simulink model "AGI_hydrogen_test9"  (R2024b)
settings: Solver=VariableStepAuto  StartTime=0.0  StopTime=Test.t_sim  RelTol=1e-3
values from neighbouring files (symbols this model uses):
  ControlSampleTime = 1/8000    (= 0.000125)    [init.m]
  f_Batt_ref = [46 47 49.9 50.1 52 53]    [init.m]
  f_PV_ref = [46 50.1 52 53]    [init.m]
  Hy_current_Ki = 20    [init.m]
  Hy_current_Kp = 0.3    [init.m]
  P_Batt_ref = [0.5 0.5 0 0 -0.5 -0.5]    [init.m]
  P_PV_ref = [1 1 1 1]    [init.m]
  PLL_Ki = 100    [init.m]
  PLL_Kp = 30    [init.m]
  Q_Batt_ref = [-0.5 -0.5 0 0.5 0.5]    [init.m]
  Q_PV_ref = [-0.5 -0.5 0 0.5 0.5]    [init.m]
  Q_ref_pu_VSM = 1    [init.m]
  S_AGI = SC_AGI    (= 25000)    [init.m]
  Test =     [S-Rocof1-OC1.mat]    (also in S-VolAngStep4-OC1.mat)
  Ts = ControlSampleTime    (= 0.000125)    [init.m]
  Ts_Control = 1e-4    (= 0.0001)    [init.m]
  Ts_Power = 5e-5    (= 5e-05)    [init.m]
  U_Batt_ref = [0.8 0.9 1 1.1 1.2]    [init.m]
  U_PV_ref = [0.8 0.9 1 1.1 1.2]    [init.m]
undefined symbols (not defined in the file or in its folder): DiscIntNeverNeededParam, Grid, Ion, L_line_PV, LCL, Lithium, sps, VSMCTRL
libraries: spsThreePhaseSeriesRLCBranchLib x10, powerlib_extras x9, spsSeriesRLCBranchLib x8, spsThreePhaseVIMeasurementLib x6, spsThreePhaseBreakerLib x6, slpidlib x6, simulink x6, spsVoltageMeasurementLib x6, FriedrichLibrary x6, spsPowerPositiveSequenceLib x5, spsUniversalBridgeLib x4, spsControlledVoltageSourceLib x4
(part 1 of 3)
settings Model: Creator=e2n051  LastModifiedBy=wshan
settings RTWCC: GPUComputeCapability=3.5

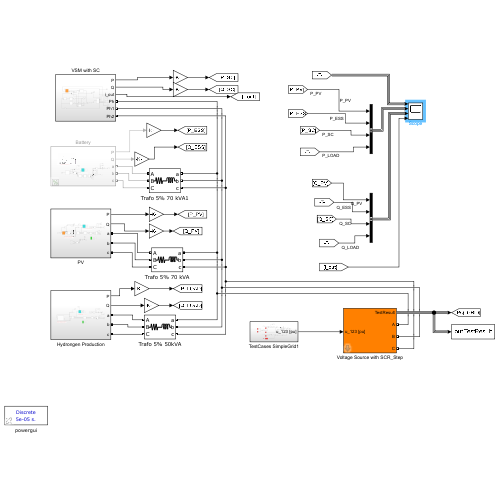
[thumbnail: Simulink's stored preview of the top-level diagram]
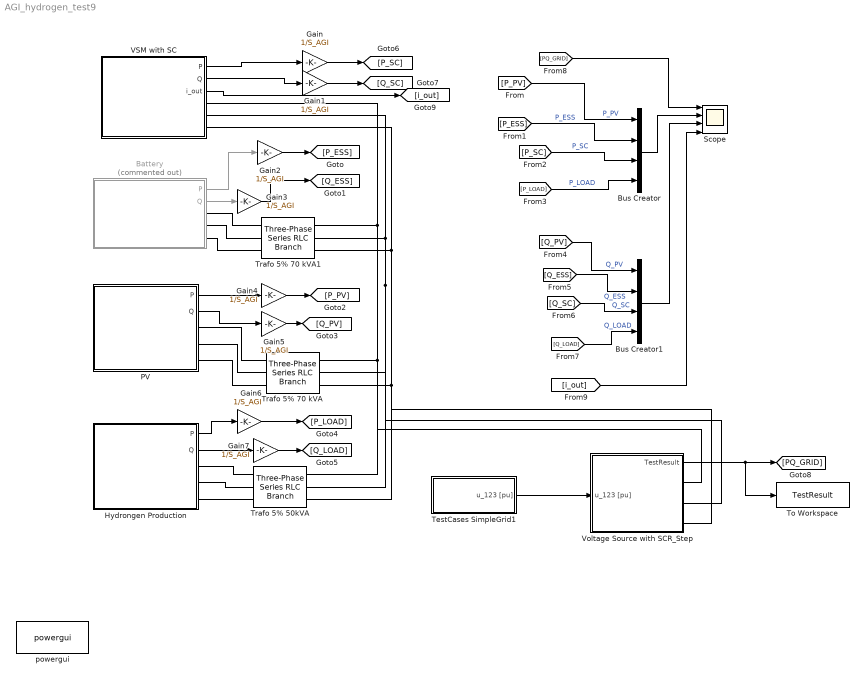
== system AGI_hydrogen_test9 ==
  Battery : Subsystem  Commented=on
  Bus Creator : BusCreator  Inputs=4
  Bus Creator1 : BusCreator  Inputs=4
  Gain{,1..7} (8 alike) : Gain  Gain=1/S_AGI
  Hydrongen Production : Subsystem
  PV : Subsystem
  Scope : Scope  NumInputPorts=4
  TestCases SimpleGrid1 : Subsystem
  To Workspace : ToWorkspace  VariableName=TestResult  SaveFormat=Timeseries  SampleTime=-1
  Trafo 5% 50kVA : spsThreePhaseSeriesRLCBranchLib/Three-Phase Series RLC Branch  LConnTagsString=A|B|C  RConnTagsString=A|B|C  BranchType=RL  Resistance=1e-3  Inductance=Test.x_trafo_pu*(400^2/(50e3))/(2*pi*50)  Capacitance=inf  Measurements=None
  Trafo 5% 70 kVA : spsThreePhaseSeriesRLCBranchLib/Three-Phase Series RLC Branch  LConnTagsString=A|B|C  RConnTagsString=A|B|C  BranchType=RL  Resistance=1e-3  Inductance=Test.x_trafo_pu*(400^2/(70e3))/(2*pi*50)  Capacitance=inf  Measurements=None
  Trafo 5% 70 kVA1 : spsThreePhaseSeriesRLCBranchLib/Three-Phase Series RLC Branch  LConnTagsString=A|B|C  RConnTagsString=A|B|C  BranchType=RL  Resistance=1e-3  Inductance=Test.x_trafo_pu*(400^2/(70e3))/(2*pi*50)  Capacitance=inf  Measurements=None
  VSM with SC : Subsystem
  Voltage Source with SCR_Step : Subsystem  mask{f0=50, Vbase=400, Sbase=S_AGI, Lpu1=Test.x_grid1, Lpu2=Test.x_grid2, Rpu1=Test.r_grid1, Rpu2=Test.r_grid2, tstep=Test.t_xgrid}
      mask prompts: f0 "Nominal Grid Frequency in Hz"; Vbase "Vbase Ph-Ph in V"; Sbase "Sbase in VA"; Lpu1 "initial X_grid in p.u."; Lpu2 "final X_grid in p.u."; Rpu1 "initial R_grid in p.u."; Rpu2 "final R_grid in p.u."; tstep "Step time grid impedance in s"
  powergui : spspowerguiLib/powergui  Priority=1  SimulationMode=Discrete  SampleTime=Ts_Power  frequency=60  Iterations=50  frequencyindice=0  Pbase=100e6  ErrMax=1e-4  UnitsV=kV  UnitsW=MW  buscounter=0  FunctionMessages=off  echomessages=off  EnableUseOfTLC=off  CurrentSourceSwitches=off  DisableSnubberDevices=off  DisableRonSwitches=off  DisableVfSwitches=off  DisplayEquations=off  AutomaticDiscreteSolvers=off  SolverType=Tustin  Interpol=off  ExternalGateDelay=off  methode=off  Ts=0  x0status=blocks  SPID=off  SwTol=0  HookPort=off  NonlinearTolerance=1e-4  nMaxIteration=100  ContinueOnMaxIteration=off  RestoreLinks=warning  ResistiveCurrentMeasurement=off  Frange=[0:2:500]  Ylog=off  Xlog=on  ShowGrid=off  save=off  variable=ZData  structure=0  ZoomFFT=on  StartTime=0.0  cycles=1  DisplayStyle=1  fundamental=60  FreqAxis=off  MaxFrequency=1000  frequencyindicesteady=1  RmsSteady=1  display=off
  wires:
  Battery/1(P) -> Gain2/1
  Battery/2(Q) -> Gain3/1
  PV/2(Q) -> Gain5/1
  PV/1(P) -> Gain4/1
  Hydrongen Production/1(P) -> Gain6/1
  Hydrongen Production/2(Q) -> Gain7/1
  VSM with SC/1(P) -> Gain/1
  [P_ESS] -> Bus Creator/2  "P_ESS"
  [P_SC] -> Bus Creator/3  "P_SC"
  Bus Creator/1 -> Scope/2
  VSM with SC/2(Q) -> Gain1/1
  [P_LOAD] -> Bus Creator/4  "P_LOAD"
  [Q_ESS] -> Bus Creator1/2  "Q_ESS"
  [Q_SC] -> Bus Creator1/3  "Q_SC"
  Bus Creator1/1 -> Scope/3
  [Q_PV] -> Bus Creator1/1  "Q_PV"
  [Q_LOAD] -> Bus Creator1/4  "Q_LOAD"
  [PQ_GRID] -> Scope/1
  VSM with SC/3(i_out) -> [i_out]
  [i_out] -> Scope/4
  Voltage Source with SCR_Step/1(TestResult) -> To Workspace/1, [PQ_GRID]
  TestCases SimpleGrid1/1(u_123 [pu]) -> Voltage Source with SCR_Step/1(u_123 [pu])
  [P_PV] -> Bus Creator/1  "P_PV"
  Gain/1 -> [P_SC]
  Gain1/1 -> [Q_SC]
  Gain2/1 -> [P_ESS]
  Gain3/1 -> [Q_ESS]
  Gain4/1 -> [P_PV]
  Gain5/1 -> [Q_PV]
  Gain6/1 -> [P_LOAD]
  Gain7/1 -> [Q_LOAD]
  connections:
  Trafo 5% 70 kVA1/RConn1 -- Voltage Source with SCR_Step/RConn1 -- Trafo 5% 50kVA/RConn1 -- Trafo 5% 70 kVA/RConn1 -- VSM with SC/RConn1
  Trafo 5% 70 kVA1/RConn3 -- Voltage Source with SCR_Step/RConn3 -- Trafo 5% 50kVA/RConn3 -- Trafo 5% 70 kVA/RConn3 -- VSM with SC/RConn3
  Trafo 5% 70 kVA1/LConn3 -- Battery/RConn3
  Trafo 5% 70 kVA1/LConn1 -- Battery/RConn1
  Trafo 5% 70 kVA1/LConn2 -- Battery/RConn2
  PV/RConn1 -- Trafo 5% 70 kVA/LConn1
  PV/RConn2 -- Trafo 5% 70 kVA/LConn2
  PV/RConn3 -- Trafo 5% 70 kVA/LConn3
  Trafo 5% 70 kVA1/RConn2 -- Voltage Source with SCR_Step/RConn2 -- Trafo 5% 50kVA/RConn2 -- Trafo 5% 70 kVA/RConn2 -- VSM with SC/RConn2
  Hydrongen Production/RConn1 -- Trafo 5% 50kVA/LConn1
  Hydrongen Production/RConn2 -- Trafo 5% 50kVA/LConn2
  Hydrongen Production/RConn3 -- Trafo 5% 50kVA/LConn3

== system AGI_hydrogen_test9/Battery ==
  note: Simple Battery Model from Matlab Standard Library:
  note: q-u-static implemented inside DC-AC converter control
  Battery : spsBatteryLib/Battery  BatType=Lithium-Ion  NomV=720  NomQ=10000  SOC=80  Batt_Tr=30  PresetModel=on  MaxQ=10000  MinV=540  FullV=838.0707  Dis_rate=4347.8261  R=0.00072  Normal_OP=9043.4783  expZone="[777.8778      491.3043]"
  L : spsThreePhaseSeriesRLCBranchLib/Three-Phase Series RLC Branch  LConnTagsString=A|B|C  RConnTagsString=A|B|C  BranchType=RL  Resistance=1e-3  Inductance=45e-6  Capacitance=inf  Measurements=None
  Mux4 : Mux  Inputs=2
  Power (Positive-Sequence) : spsPowerPositiveSequenceLib/Power (Positive-Sequence)  Freq=50  Vinit=[20200 0]  Iinit=[12.3 0]  Ts=Ts_Control
  Scope{,1..4} (5 alike) : Scope
  Three-Phase V-I Measurement : spsThreePhaseVIMeasurementLib/Three-Phase V-I Measurement  VoltageMeasurement=phase-to-ground  SetLabelV=off  LabelV=Vabc  Vpu=off  VpuLL=off  CurrentMeasurement=yes  SetLabelI=off  LabelI=Iabc  Ipu=off  Pbase=100e6  Vbase=500e3  OutputType=Complex  PhasorSimulation=off  PSBequivalent=0
  Three-Phase Breaker : spsThreePhaseBreakerLib/Three-Phase Breaker  InitialState=closed  SwitchA=on  SwitchB=on  SwitchC=on  SwitchTimes=100  External=off  BreakerResistance=0.0001  SnubberResistance=1e6  SnubberCapacitance=inf  Measurements=None
  VSC (Average Model)1 : spsUniversalBridgeLib/Universal Bridge  Arms=3  SnubberResistance=1e5  SnubberCapacitance=inf  Device=Average-model based VSC  Ron=1e-3  Lon=0  ForwardVoltages="[  0  0  ]"  ForwardVoltage=0  GTOparameters=[ 10e-6 , 20e-6 ]  IGBTparameters=[ 1e-6 , 2e-6 ]  Measurements=None  Measurements_2=None  converterType=Rectifier
  VSC Control1 : Subsystem  mask(VSC Main Controller){nom=[ 69e3  50], Vnom=[ 400 400 ], Vnom_dc=700, RLxfo=[0.002  0.06 ]*0, RLchoke=[1e-3  45e-6  ], K_VDCreg=[1  400]*10, K_Ireg=[0.3/4 20/4]*4, Ts=Ts_Control}
      mask prompts: nom "Nominal power and frequency [ Pnom(VA)  Fnom(Hz) ]:"; Vnom "Nominal primary and secondary voltages (Vrms LL) [ Vnom_prim   Vnom_sec ]:"; Vnom_dc "Nominal DC bus voltage (V):"; RLxfo "Total transformer leakage impedance (pu/Pnom) [ Rxfo  Lxf ]"; RLchoke "Choke impedance [ R(ohm) L(H) ]"; K_VDCreg "VDC regultator gains [ Kp  Ki ]:"; K_Ireg "Current regulator gains [ Kp  Ki ]:"; Ts "Sample time"
      mask init:
      | Pnom=nom(1);
      | Fnom=nom(2);
      | Vnom_prim=Vnom(1);
      | Vnom_sec=Vnom(2);
      | Zbase=Vnom_sec^2/Pnom;
      | Rtot_pu=RLxfo(1) + RLchoke(1)/Zbase;
      | Ltot_pu=RLxfo(2) + RLchoke(2)/(Zbase/(2*pi*Fnom));
      | Kp_VDCreg=K_VDCreg(1);
      | Ki_VDCreg=K_VDCreg(2);
      | Kp_Ireg=K_Ireg(1);
      | Ki_Ireg=K_Ireg(2);
      | Vdc_ref=Vnom_dc;
  Vdc 1 : spsVoltageMeasurementLib/Voltage Measurement  Tag=PoWeRsYsTeMmEaSuReMeNt  PhasorSimulation=off  OutputType=Magnitude  PSBequivalent=0
  to-Kva : Gain  Gain=1/1000
  a : PMIOPort  Side=Right
  b : PMIOPort  Port=2  Side=Right
  c : PMIOPort  Port=3  Side=Right
  P : Outport
  Q : Outport  Port=2
  wires:
  Battery/1 -> Scope/1
  VSC Control1/1(Uref) -> VSC (Average Model)1/1
  Vdc 1/1 -> [Vdc], Scope2/1
  [Igrid] -> VSC Control1/2(I)
  [Vgrid] -> VSC Control1/1(V)
  Three-Phase V-I Measurement/1 -> Scope3/1, Power (Positive-Sequence)/1, [Vgrid]
  Three-Phase V-I Measurement/2 -> [Igrid], Power (Positive-Sequence)/2, Scope4/1
  Power (Positive-Sequence)/2 -> Q/1, Mux4/2
  to-Kva/1 -> Scope1/1  "PQ (kVA)"
  Mux4/1 -> to-Kva/1
  Power (Positive-Sequence)/1 -> P/1, Mux4/1
  connections:
  Battery/LConn2 -- Vdc 1/LConn2 -- VSC (Average Model)1/RConn2
  VSC (Average Model)1/RConn1 -- Vdc 1/LConn1 -- Battery/LConn1
  L/RConn3 -- Three-Phase V-I Measurement/LConn3
  VSC (Average Model)1/LConn2 -- Three-Phase Breaker/LConn2
  L/LConn2 -- Three-Phase Breaker/RConn2
  L/LConn3 -- Three-Phase Breaker/RConn3
  a/RConn1 -- Three-Phase V-I Measurement/RConn1
  Three-Phase Breaker/RConn1 -- L/LConn1
  Three-Phase V-I Measurement/LConn2 -- L/RConn2
  VSC (Average Model)1/LConn3 -- Three-Phase Breaker/LConn3
  Three-Phase V-I Measurement/RConn3 -- c/RConn1
  VSC (Average Model)1/LConn1 -- Three-Phase Breaker/LConn1
  Three-Phase V-I Measurement/RConn2 -- b/RConn1
  L/RConn1 -- Three-Phase V-I Measurement/LConn1

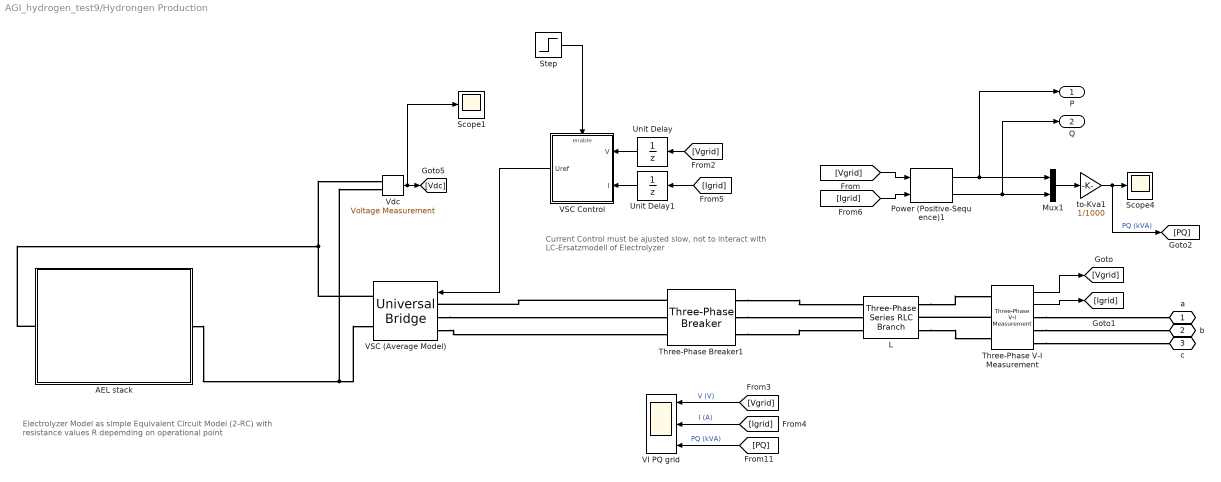
== system AGI_hydrogen_test9/Hydrongen Production ==
  note: Current Control must be ajusted slow, not to interact with
      | LC-Ersatzmodell of Electrolyzer
  note: Electrolyzer Model as simple Equivalent Circuit Model (2-RC)
      | with resistance values R depemding on operational point
  AEL stack : Subsystem  mask{A_cell=300, N_cell=500, P_min_share=10, P_max_share=100, i_nom=0.165, ResultPIV=|, R_cell_ohm=0.89, Ca=1, Cc=100, a=0.04, c=0.12, i0=1.2e-4, V_rev=1.26, I0_a=1650, I0_c=1650, V0_a_cell=0.25, V0_c_cell=0.25}
      mask ResultPIV=|
      | Nominal power in kW: 47.25
      | Operating power range in kW: 4.72 - 47.25
      |
      | Nominal voltage in V: 954.49
      | Nominal current in A: 49.50
      mask prompts: A_cell "Cell active area A_cell in cm^2"; N_cell "Number of cells N_cell"; P_min_share "Minimum power in %"; P_max_share "Maximum power in %"; i_nom "Nominal current desnity in A/cm^2"; R_cell_ohm "Ohmic cell resistance in Ohm/cm^2"; Ca "Anode cell capacity in mF/cm^2"; Cc "Cathode cell capacity in mF/cm^2"; a "Anode tafel slope in V/dec"; c "Cathode tafel slope in V/dec"; i0 "Exchange current density in A/cm^2"; V_rev "Reversible cell voltage in V"; I0_a "Initial resistor current at anode"; I0_c "Initial resistor current at cathode"; V0_a_cell "Initial capacitor anode cell voltage in V"; V0_c_cell "Initial capacitor cathode cell voltage in V"
      mask DialogControl PIV_calc Prompt: Get: power / voltage / current
      mask DialogControl PIV_calc Tooltip: Press button for calculation
  L : spsThreePhaseSeriesRLCBranchLib/Three-Phase Series RLC Branch  LConnTagsString=A|B|C  RConnTagsString=A|B|C  BranchType=RL  Resistance=1e-3  Inductance=45e-6  Capacitance=inf  Measurements=None
  Mux1 : Mux  Inputs=2
  Power (Positive-Sequence)1 : spsPowerPositiveSequenceLib/Power (Positive-Sequence)  Freq=60  Vinit=[20200 0]  Iinit=[12.3 0]  Ts=Ts_Control
  Scope1 : Scope
  Scope4 : Scope
  Step : Step  Time=0  SampleTime=0
  Three-Phase V-I Measurement : spsThreePhaseVIMeasurementLib/Three-Phase V-I Measurement  VoltageMeasurement=phase-to-ground  SetLabelV=off  LabelV=Vabc  Vpu=off  VpuLL=off  CurrentMeasurement=yes  SetLabelI=off  LabelI=Iabc  Ipu=off  Pbase=100e6  Vbase=500e3  OutputType=Complex  PhasorSimulation=off  PSBequivalent=0
  Three-Phase Breaker1 : spsThreePhaseBreakerLib/Three-Phase Breaker  InitialState=open  SwitchA=on  SwitchB=on  SwitchC=on  SwitchTimes=0  External=off  BreakerResistance=0.0001  SnubberResistance=1e6  SnubberCapacitance=inf  Measurements=None
  Unit Delay : UnitDelay  SampleTime=Ts  HasFrameUpgradeWarning=on
  Unit Delay1 : UnitDelay  SampleTime=Ts  HasFrameUpgradeWarning=on
  VI PQ grid : Scope  NumInputPorts=3
  VSC (Average Model) : spsUniversalBridgeLib/Universal Bridge  Arms=3  SnubberResistance=1e5  SnubberCapacitance=inf  Device=Average-model based VSC  Ron=1e-3  Lon=0  ForwardVoltages="[  0  0  ]"  ForwardVoltage=0  GTOparameters=[ 10e-6 , 20e-6 ]  IGBTparameters=[ 1e-6 , 2e-6 ]  Measurements=None  Measurements_2=None  converterType=Rectifier
  VSC Control : Subsystem  mask(VSC Main Controller){nom=[ 50e3  50 ], Vnom=[ 400 400 ], Vnom_dc=720, RLxfo=[0.002  0.06 ]*0, RLchoke=[1e-3  45e-6  ], K_VDCreg=[7  800], K_Ireg=[Hy_current_Kp  Hy_current_Ki], Ts=Ts_Control}
      mask prompts: nom "Nominal power and frequency [ Pnom(VA)  Fnom(Hz) ]:"; Vnom "Nominal primary and secondary voltages (Vrms LL) [ Vnom_prim   Vnom_sec ]:"; Vnom_dc "Nominal DC bus voltage (V):"; RLxfo "Total transformer leakage impedance (pu/Pnom) [ Rxfo  Lxf ]"; RLchoke "Choke impedance [ R(ohm) L(H) ]"; K_VDCreg "VDC regultator gains [ Kp  Ki ]:"; K_Ireg "Current regulator gains [ Kp  Ki ]:"; Ts "Sample time"
      mask init: same as AGI_hydrogen_test9/Battery/VSC Control1
  "Vdc " : spsVoltageMeasurementLib/Voltage Measurement  Tag=PoWeRsYsTeMmEaSuReMeNt  PhasorSimulation=off  OutputType=Magnitude  PSBequivalent=0
  to-Kva1 : Gain  Gain=1/1000
  a : PMIOPort  Side=Right
  b : PMIOPort  Port=2  Side=Right
  c : PMIOPort  Port=3  Side=Right
  P : Outport
  Q : Outport  Port=2
  wires:
  Three-Phase V-I Measurement/2 -> [Igrid]
  Three-Phase V-I Measurement/1 -> [Vgrid]
  [PQ] -> VI PQ grid/3  "PQ (kVA)"
  [Vgrid] -> VI PQ grid/1  "V (V)"
  to-Kva1/1 -> [PQ], Scope4/1  "PQ (kVA)"
  [Igrid] -> VI PQ grid/2  "I (A)"
  VSC Control/1(Uref) -> VSC (Average Model)/1
  Step/1 -> VSC Control/Enable
  "Vdc "/1 -> Scope1/1, [Vdc]
  [Vgrid] -> Unit Delay/1
  [Vgrid] -> Power (Positive-Sequence)1/1
  Power (Positive-Sequence)1/2 -> Q/1, Mux1/2
  Mux1/1 -> to-Kva1/1
  [Igrid] -> Power (Positive-Sequence)1/2
  Power (Positive-Sequence)1/1 -> P/1, Mux1/1
  Unit Delay/1 -> VSC Control/1(V)
  [Igrid] -> Unit Delay1/1
  Unit Delay1/1 -> VSC Control/2(I)
  connections:
  Three-Phase V-I Measurement/RConn3 -- c/RConn1
  Three-Phase V-I Measurement/RConn1 -- a/RConn1
  Three-Phase V-I Measurement/RConn2 -- b/RConn1
  L/RConn3 -- Three-Phase V-I Measurement/LConn3
  L/RConn1 -- Three-Phase V-I Measurement/LConn1
  Three-Phase V-I Measurement/LConn2 -- L/RConn2
  Three-Phase Breaker1/RConn1 -- L/LConn1
  Three-Phase Breaker1/RConn3 -- L/LConn3
  Three-Phase Breaker1/RConn2 -- L/LConn2
  AEL stack/RConn1 -- "Vdc "/LConn2 -- VSC (Average Model)/RConn2
  VSC (Average Model)/LConn3 -- Three-Phase Breaker1/LConn3
  VSC (Average Model)/LConn2 -- Three-Phase Breaker1/LConn2
  Three-Phase Breaker1/LConn1 -- VSC (Average Model)/LConn1
  AEL stack/LConn1 -- VSC (Average Model)/RConn1 -- "Vdc "/LConn1

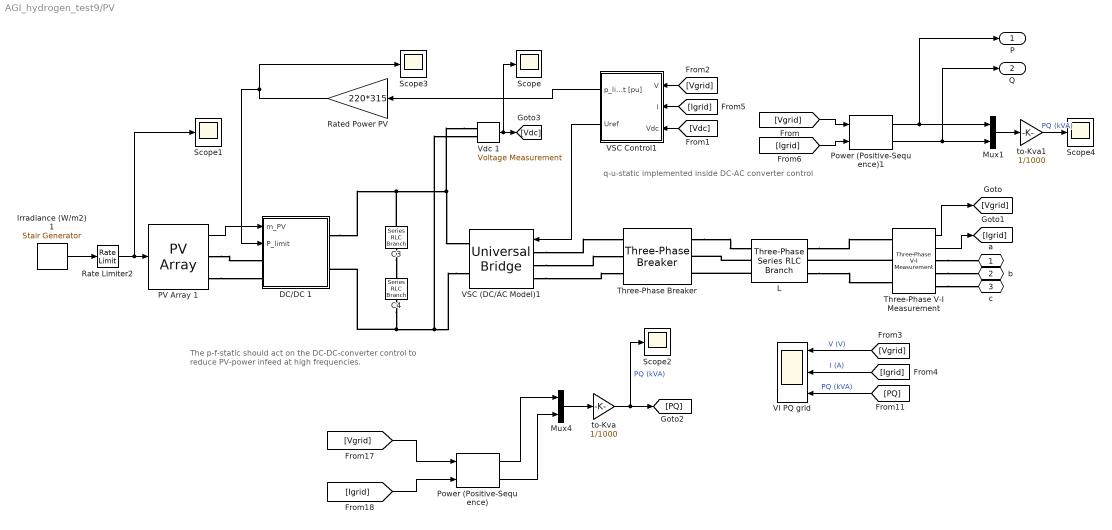
== system AGI_hydrogen_test9/PV ==
  note: The p-f-static should act on the DC-DC-converter control
      | to reduce PV-power infeed at high frequencies.
  note: q-u-static implemented inside DC-AC converter control
  C3 : spsSeriesRLCBranchLib/Series RLC Branch  LConnTagsString=__new0  RConnTagsString=__new0  BranchType=C  Resistance=1.0  Inductance=1.0  SetiL0=off  InitialCurrent=0  Capacitance=100e-3  Setx0=on  InitialVoltage=350  Measurements=None
  C4 : spsSeriesRLCBranchLib/Series RLC Branch  LConnTagsString=__new0  RConnTagsString=__new0  BranchType=C  Resistance=1.0  Inductance=1.0  SetiL0=off  InitialCurrent=0  Capacitance=100e-3  Setx0=on  InitialVoltage=350  Measurements=None
  DC/DC 1 : Subsystem
  Irradiance (W/m2) 1 : spsStairGeneratorLib/Stair Generator  t=[0, 0.5, 2.3]  e=[1,1.0, 1.0]*1000  Ts=Ts_Power
  L : spsThreePhaseSeriesRLCBranchLib/Three-Phase Series RLC Branch  LConnTagsString=A|B|C  RConnTagsString=A|B|C  BranchType=RL  Resistance=1e-3  Inductance=45e-6  Capacitance=inf  Measurements=None
  Mux1 : Mux  Inputs=2
  Mux4 : Mux  Inputs=2
  PV Array 1 : spsPVArrayLib/PV Array  Npar=220/7  Nser=7  PlotType=array @ 1000 W/m2 & specified temperatures  S_vec="[ 1000  500  100 ]"  Temp_C_vec="[ 45 25  ]"  ModuleName=SunPower SPR-315E-WHT-D  PlotWhenSelected=off  Pm=315.072  Ncell=96  Voc=64.6  Isc=6.14  Vm=54.7  Im=5.76  beta_Voc_pc=-0.2727  alpha_Isc_pc=0.061743  beta_Voc=-0.17616  alpha_Isc=0.003791  IL=6.1461  I0=6.5067e-12  nI=0.95071  Rsh=430.0666  Rs=0.43041  RobustModel=on  RobustCellTemperature=40  BAL=off  Tc=1e-6  Tfilter=5e-5
  Power (Positive-Sequence) : spsPowerPositiveSequenceLib/Power (Positive-Sequence)  Freq=60  Vinit=[20200 0]  Iinit=[12.3 0]  Ts=Ts_Control
  Power (Positive-Sequence)1 : spsPowerPositiveSequenceLib/Power (Positive-Sequence)  Freq=60  Vinit=[20200 0]  Iinit=[12.3 0]  Ts=Ts_Control
  Rate Limiter2 : RateLimiter  RisingSlewLimit=8000  FallingSlewLimit=-8000  SampleTimeMode=inherited  InitialCondition=1000
  Rated Power PV : Gain  Gain=220*315
  Scope{,1..4} (5 alike) : Scope
  Three-Phase V-I Measurement : spsThreePhaseVIMeasurementLib/Three-Phase V-I Measurement  VoltageMeasurement=phase-to-ground  SetLabelV=off  LabelV=Vabc  Vpu=off  VpuLL=off  CurrentMeasurement=yes  SetLabelI=off  LabelI=Iabc  Ipu=off  Pbase=100e6  Vbase=500e3  OutputType=Complex  PhasorSimulation=off  PSBequivalent=0
  Three-Phase Breaker : spsThreePhaseBreakerLib/Three-Phase Breaker  InitialState=open  SwitchA=on  SwitchB=on  SwitchC=on  SwitchTimes=0  External=off  BreakerResistance=0.0001  SnubberResistance=1e6  SnubberCapacitance=inf  Measurements=None
  VI PQ grid : Scope  NumInputPorts=3
  VSC (DC/AC Model)1 : spsUniversalBridgeLib/Universal Bridge  Arms=3  SnubberResistance=1e5  SnubberCapacitance=inf  Device=Average-model based VSC  Ron=1e-3  Lon=0  ForwardVoltages="[  0  0  ]"  ForwardVoltage=0  GTOparameters=[ 10e-6 , 20e-6 ]  IGBTparameters=[ 1e-6 , 2e-6 ]  Measurements=None  Measurements_2=None  converterType=Rectifier
  VSC Control1 : Subsystem  mask(VSC Main Controller){nom=[ 69e3  50], Vnom=[ 400 400 ], Vnom_dc=700, RLxfo=[0.002  0.06 ]*0, RLchoke=[1e-3  45e-6  ], K_VDCreg=[2  400]*10, K_Ireg=[0.3 20], Ts=Ts_Control}
      mask prompts: nom "Nominal power and frequency [ Pnom(VA)  Fnom(Hz) ]:"; Vnom "Nominal primary and secondary voltages (Vrms LL) [ Vnom_prim   Vnom_sec ]:"; Vnom_dc "Nominal DC bus voltage (V):"; RLxfo "Total transformer leakage impedance (pu/Pnom) [ Rxfo  Lxf ]"; RLchoke "Choke impedance [ R(ohm) L(H) ]"; K_VDCreg "VDC regultator gains [ Kp  Ki ]:"; K_Ireg "Current regulator gains [ Kp  Ki ]:"; Ts "Sample time"
      mask init: same as AGI_hydrogen_test9/Battery/VSC Control1
  Vdc 1 : spsVoltageMeasurementLib/Voltage Measurement  Tag=PoWeRsYsTeMmEaSuReMeNt  PhasorSimulation=off  OutputType=Magnitude  PSBequivalent=0
  to-Kva : Gain  Gain=1/1000
  to-Kva1 : Gain  Gain=1/1000
  a : PMIOPort  Side=Right
  b : PMIOPort  Port=2  Side=Right
  c : PMIOPort  Port=3  Side=Right
  P : Outport
  Q : Outport  Port=2
  wires:
  [Igrid] -> Power (Positive-Sequence)/2
  [Igrid] -> VI PQ grid/2  "I (A)"
  to-Kva/1 -> Scope2/1, [PQ]  "PQ (kVA)"
  [Vgrid] -> VI PQ grid/1  "V (V)"
  Mux4/1 -> to-Kva/1
  [PQ] -> VI PQ grid/3  "PQ (kVA)"
  [Vgrid] -> Power (Positive-Sequence)/1
  Power (Positive-Sequence)/1 -> Mux4/1
  Power (Positive-Sequence)/2 -> Mux4/2
  Three-Phase V-I Measurement/1 -> [Vgrid]
  Three-Phase V-I Measurement/2 -> [Igrid]
  VSC Control1/2(Uref) -> VSC (DC/AC Model)1/1
  Irradiance (W/m2) 1/1 -> Rate Limiter2/1
  [Vdc] -> VSC Control1/3(Vdc)
  PV Array 1/1 -> DC/DC 1/1(m_PV)
  Vdc 1/1 -> Scope/1, [Vdc]
  [Igrid] -> VSC Control1/2(I)
  [Vgrid] -> VSC Control1/1(V)
  Rate Limiter2/1 -> Scope1/1, PV Array 1/1
  VSC Control1/1(p_limit [pu]) -> Rated Power PV/1
  Rated Power PV/1 -> DC/DC 1/2(P_limit), Scope3/1
  Mux1/1 -> to-Kva1/1
  Power (Positive-Sequence)1/2 -> Q/1, Mux1/2
  Power (Positive-Sequence)1/1 -> P/1, Mux1/1
  to-Kva1/1 -> Scope4/1  "PQ (kVA)"
  [Vgrid] -> Power (Positive-Sequence)1/1
  [Igrid] -> Power (Positive-Sequence)1/2
  connections:
  VSC (DC/AC Model)1/LConn3 -- Three-Phase Breaker/LConn3
  L/LConn2 -- Three-Phase Breaker/RConn2
  VSC (DC/AC Model)1/LConn1 -- Three-Phase Breaker/LConn1
  L/LConn3 -- Three-Phase Breaker/RConn3
  Three-Phase Breaker/RConn1 -- L/LConn1
  VSC (DC/AC Model)1/LConn2 -- Three-Phase Breaker/LConn2
  Three-Phase V-I Measurement/LConn2 -- L/RConn2
  L/RConn1 -- Three-Phase V-I Measurement/LConn1
  L/RConn3 -- Three-Phase V-I Measurement/LConn3
  Three-Phase V-I Measurement/RConn2 -- b/RConn1
  Three-Phase V-I Measurement/RConn1 -- a/RConn1
  Three-Phase V-I Measurement/RConn3 -- c/RConn1
  Vdc 1/LConn1 -- C3/LConn1 -- DC/DC 1/RConn1 -- VSC (DC/AC Model)1/RConn1
  VSC (DC/AC Model)1/RConn2 -- C4/RConn1 -- DC/DC 1/RConn2 -- Vdc 1/LConn2
  C3/RConn1 -- C4/LConn1
  PV Array 1/RConn2 -- DC/DC 1/LConn2
  PV Array 1/RConn1 -- DC/DC 1/LConn1

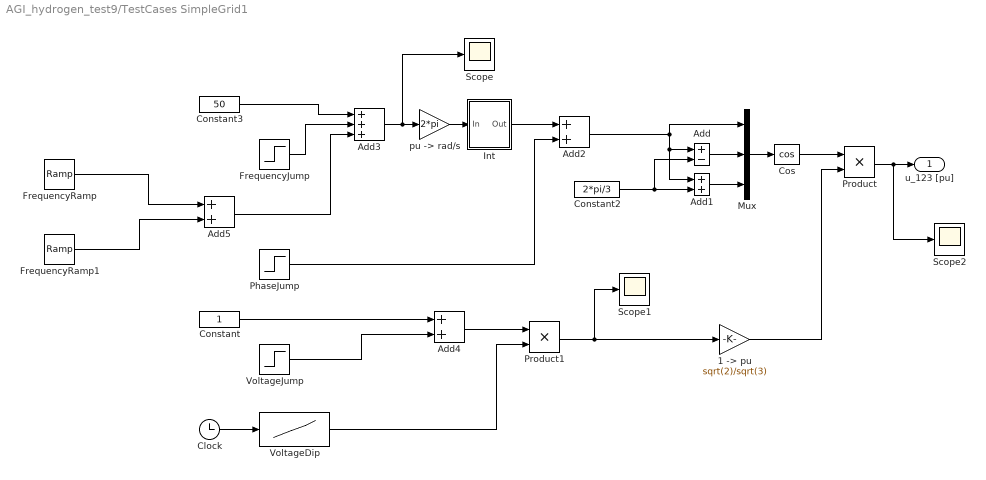
== system AGI_hydrogen_test9/TestCases SimpleGrid1 ==
  "1 -> pu" : Gain  Gain=sqrt(2)/sqrt(3)
  Add : Sum  Inputs=+-
  Add{1..2,4..5} (4 alike) : Sum
  Add3 : Sum  Inputs=+++
  Clock : Clock
  Constant : Constant
  Constant2 : Constant  Value=2*pi/3
  Constant3 : Constant  Value=50
  Cos : Trigonometry  Operator=cos
  FrequencyJump : Step  Time=Test.t_start  After=Test.delta_f  SampleTime=0
  FrequencyRamp : simulink/Sources/Ramp  slope=Test.ramp_f_ROCOF  start=Test.t_start  InitialOutput=0
  FrequencyRamp1 : simulink/Sources/Ramp  slope=-Test.ramp_f_ROCOF  start=Test.t_start+Test.ramp_f_duration  InitialOutput=0
  Int : Subsystem
  Mux : Mux  Inputs=3
  PhaseJump : Step  Time=Test.t_start  After=Test.delta_phi/180*pi  SampleTime=0
  Product : Product
  Product1 : Product
  Scope : Scope
  Scope1 : Scope
  Scope2 : Scope
  VoltageDip : Lookup_n-D  NumberOfTableDimensions=1  BreakpointsForDimension1=[-1 0 0.01 0.15 0.16 2]+Test.t_start  Table=[1 1 1 1 1 1] - Test.delta_u_fault*[0 0 1 1 0 0]  InternalRulePriority=Speed  RndMeth=Simplest
  VoltageJump : Step  Time=Test.t_start  After=Test.delta_u  SampleTime=0
  "pu -> rad/s" : Gain  Gain=2*pi
  u_123 [pu] : Outport
  wires:
  Clock/1 -> VoltageDip/1
  Constant/1 -> Add4/1
  PhaseJump/1 -> Add2/2
  VoltageJump/1 -> Add4/2
  Add1/1 -> Mux/3
  Product/1 -> Scope2/1, u_123 [pu]/1
  "pu -> rad/s"/1 -> Int/1(In)
  Constant2/1 -> Add/2, Add1/2
  Cos/1 -> Product/1
  Add/1 -> Mux/2
  Mux/1 -> Cos/1
  Int/1(Out) -> Add2/1
  Add4/1 -> Product1/1
  Add3/1 -> Scope/1, "pu -> rad/s"/1
  Add2/1 -> Mux/1, Add1/1, Add/1
  Product1/1 -> "1 -> pu"/1, Scope1/1
  Constant3/1 -> Add3/1
  FrequencyJump/1 -> Add3/2
  VoltageDip/1 -> Product1/2
  "1 -> pu"/1 -> Product/2
  FrequencyRamp/1 -> Add5/1
  FrequencyRamp1/1 -> Add5/2
  Add5/1 -> Add3/3

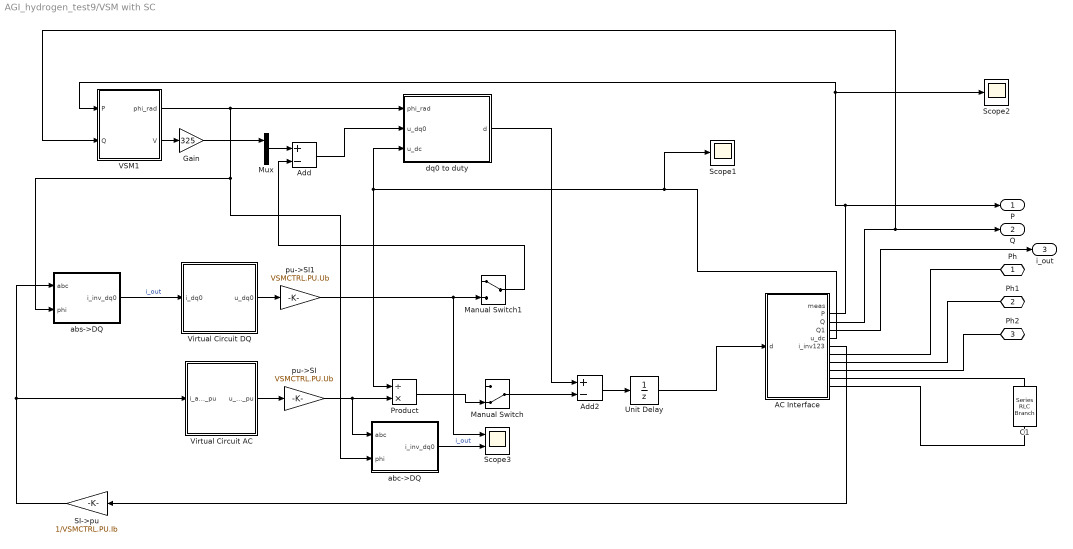
== system AGI_hydrogen_test9/VSM with SC ==
  AC Interface : Subsystem
  Add : Sum  Inputs=+-
  Add2 : Sum  Inputs=+-
  C1 : spsSeriesRLCBranchLib/Series RLC Branch  LConnTagsString=__new0  RConnTagsString=__new0  BranchType=C  Resistance=0.001  Inductance=L_line_PV  SetiL0=off  InitialCurrent=0  Capacitance=0.63  Setx0=on  InitialVoltage=800  Measurements=Branch voltage
  Gain : Gain  Gain=325
  Manual Switch : ManualSwitch  CurrentSetting=0
  Manual Switch1 : ManualSwitch
  Mux : Mux  Inputs=3
  Product : Product  Inputs=/*
  SI->pu : Gain  Gain=1/VSMCTRL.PU.Ib
  Scope1 : Scope
  Scope2 : Scope
  Scope3 : Scope  NumInputPorts=2
  Unit Delay : UnitDelay  SampleTime=-1  HasFrameUpgradeWarning=on
  VSM1 : Subsystem
  Virtual Circuit AC : Subsystem  AncestorBlock=ControLibrary/Virtual Circuit
      settings: LibrarySourceBlock=ControLibrary/Virtual Circuit
  Virtual Circuit DQ : Subsystem  AncestorBlock=ControLibrary/Virtual Circuit
      settings: LibrarySourceBlock=ControLibrary/Virtual Circuit
  abc->DQ : Subsystem
  abs->DQ : Subsystem
  dq0 to duty : Subsystem
  pu->SI : Gain  Gain=VSMCTRL.PU.Ub
  pu->SI1 : Gain  Gain=VSMCTRL.PU.Ub
  Ph : PMIOPort  Side=Right
  Ph1 : PMIOPort  Port=2  Side=Right
  Ph2 : PMIOPort  Port=3  Side=Right
  P : Outport
  Q : Outport  Port=2
  i_out : Outport  Port=3
  wires:
  AC Interface/2(P) -> VSM1/1(P), Scope2/1, P/1
  AC Interface/3(Q) -> VSM1/2(Q), Q/1
  AC Interface/4(Q1) -> i_out/1
  VSM1/1(phi_rad) -> abs->DQ/2(phi), abc->DQ/2(phi), dq0 to duty/1(phi_rad)
  AC Interface/5(u_dc) -> Scope1/1, Product/1, dq0 to duty/3(u_dc)
  Unit Delay/1 -> AC Interface/1(d)
  VSM1/2(V) -> Gain/1
  Gain/1 -> Mux/1
  Mux/1 -> Add/1
  Add/1 -> dq0 to duty/2(u_dq0)
  abs->DQ/1(i_inv_dq0) -> Virtual Circuit DQ/1(i_dq0)  "i_out"
  AC Interface/6(i_inv123) -> SI->pu/1
  SI->pu/1 -> Virtual Circuit AC/1(i_abc_pu), abs->DQ/1(abc)
  Virtual Circuit DQ/1(" u_dq0") -> pu->SI1/1
  pu->SI1/1 -> Manual Switch1/2, Scope3/1
  Virtual Circuit AC/1(" u_abc_pu") -> pu->SI/1
  pu->SI/1 -> Product/2, abc->DQ/1(abc)
  Add2/1 -> Unit Delay/1
  dq0 to duty/1(d) -> Add2/1
  abc->DQ/1(i_inv_dq0) -> Scope3/2  "i_out"
  Product/1 -> Manual Switch/2
  Manual Switch/1 -> Add2/2
  Manual Switch1/1 -> Add/2
  connections:
  AC Interface/RConn1 -- Ph/RConn1
  AC Interface/RConn2 -- Ph1/RConn1
  AC Interface/RConn3 -- Ph2/RConn1
  AC Interface/RConn4 -- C1/LConn1
  AC Interface/RConn5 -- C1/RConn1

== system AGI_hydrogen_test9/Voltage Source with SCR_Step ==
  u_123 [pu] : Inport
  Bus Creator2 : BusCreator  Inputs=2
  Demux1 : Demux  Outputs=3
  Ea1 : spsControlledVoltageSourceLib/Controlled Voltage Source  Initialize=off  Source_Type=AC  Amplitude=0  Phase=0  Frequency=0  Measurements=None
  Eb1 : spsControlledVoltageSourceLib/Controlled Voltage Source  Initialize=off  Source_Type=AC  Amplitude=0  Phase=0  Frequency=0  Measurements=None
  Ec1 : spsControlledVoltageSourceLib/Controlled Voltage Source  Initialize=off  Source_Type=AC  Amplitude=0  Phase=0  Frequency=0  Measurements=None
  Gain : Gain  Gain=1/Sbase
  Gain1 : Gain  Gain=1/Sbase
  Ground2 : spsGroundLib/Ground  LConnTagsString=a
  L1 : spsThreePhaseSeriesRLCBranchLib/Three-Phase Series RLC Branch  LConnTagsString=A|B|C  RConnTagsString=A|B|C  BranchType=RL  Resistance=Rpu1*(Vbase^2/Sbase)  Inductance=Lpu1*(Vbase^2/Sbase/(2*pi*f0))  Capacitance=inf  Measurements=None
  L4 : spsThreePhaseSeriesRLCBranchLib/Three-Phase Series RLC Branch  LConnTagsString=A|B|C  RConnTagsString=A|B|C  BranchType=RL  Resistance=(Rpu2-Rpu1)*(Vbase^2/Sbase)  Inductance=(Lpu2-Lpu1)*(Vbase^2/Sbase/(2*pi*f0))  Capacitance=inf  Measurements=None
  Power Measurement (Three-Phase) : eePowerMeasurement/Power Measurement (Three-Phase)  LabelModeActiveChoice=Continuous  F=f0  K=[1]  Seq=Positive  Ts=0
  Three-Phase V-I Measurement : spsThreePhaseVIMeasurementLib/Three-Phase V-I Measurement  VoltageMeasurement=phase-to-ground  SetLabelV=off  LabelV=Vabc  Vpu=off  VpuLL=off  CurrentMeasurement=yes  SetLabelI=off  LabelI=Iabc  Ipu=off  Pbase=100e6  Vbase=500e3  OutputType=Complex  PhasorSimulation=off  PSBequivalent=0
  Three-Phase Breaker : spsThreePhaseBreakerLib/Three-Phase Breaker  InitialState=closed  SwitchA=on  SwitchB=on  SwitchC=on  SwitchTimes=tstep  External=off  BreakerResistance=0.0001  SnubberResistance=1e6  SnubberCapacitance=inf  Measurements=None
  "pu -> V" : Gain  Gain=Vbase
  A : PMIOPort  Side=Right
  B : PMIOPort  Port=2  Side=Right
  C : PMIOPort  Port=3  Side=Right
  TestResult : Outport
  wires:
  Demux1/1 -> Ea1/1
  Demux1/3 -> Ec1/1
  Demux1/2 -> Eb1/1
  u_123 [pu]/1 -> "pu -> V"/1
  Bus Creator2/1 -> TestResult/1
  Power Measurement (Three-Phase)/2 -> Gain1/1  "Q_GRID"
  Power Measurement (Three-Phase)/1 -> Gain/1  "P_GRID"
  Three-Phase V-I Measurement/1 -> Power Measurement (Three-Phase)/1
  Three-Phase V-I Measurement/2 -> Power Measurement (Three-Phase)/2
  Gain/1 -> Bus Creator2/1  "P_GRID_pu"
  Gain1/1 -> Bus Creator2/2  "Q_GRID_pu"
  "pu -> V"/1 -> Demux1/1
  connections:
  Eb1/LConn1 -- Ec1/LConn1 -- Ground2/LConn1 -- Ea1/LConn1
  L4/RConn1 -- Three-Phase Breaker/RConn1 -- Three-Phase V-I Measurement/RConn1
  Three-Phase V-I Measurement/RConn2 -- Three-Phase Breaker/RConn2 -- L4/RConn2
  Three-Phase V-I Measurement/RConn3 -- Three-Phase Breaker/RConn3 -- L4/RConn3
  Three-Phase Breaker/LConn1 -- L1/RConn1 -- L4/LConn1
  Three-Phase Breaker/LConn2 -- L1/RConn2 -- L4/LConn2
  Three-Phase Breaker/LConn3 -- L1/RConn3 -- L4/LConn3
  Ea1/RConn1 -- L1/LConn1
  Eb1/RConn1 -- L1/LConn2
  Ec1/RConn1 -- L1/LConn3
  Three-Phase V-I Measurement/LConn1 -- A/RConn1
  Three-Phase V-I Measurement/LConn2 -- B/RConn1
  Three-Phase V-I Measurement/LConn3 -- C/RConn1

== system AGI_hydrogen_test9/Battery/VSC Control1 ==
  note: VSC Main Controller
  V : Inport  PortDimensions=3
  I : Inport  Port=2  PortDimensions=3
  Converter Current Limit pu : Constant  Value=1.5
  Current Regulator : Subsystem
  Mux1 : Mux  Inputs=2
  Mux2 : Mux  Inputs=2
  PLL & Measurements : Subsystem
  Saturation : Saturate  UpperLimit=2  LowerLimit=-2
  Saturation1 : Saturate  UpperLimit=2  LowerLimit=-2
  Scope1 : Scope
  Scope3 : Scope
  Selector : Selector  InputPortWidth=2  IndexOptions=Index vector (dialog)  Indices=[1]  OutputSizes=1
  Selector1 : Selector  InputPortWidth=2  IndexOptions=Index vector (dialog)  Indices=[1]  OutputSizes=1
  Selector2 : Selector  InputPortWidth=2  IndexOptions=Index vector (dialog)  Indices=[2]  OutputSizes=1
  Selector3 : Selector  InputPortWidth=2  IndexOptions=Index vector (dialog)  Indices=[2]  OutputSizes=1
  Uabc_ref Generation max (m) = 1 : Subsystem
  Unit Delay : UnitDelay  SampleTime=Ts_Control  HasFrameUpgradeWarning=on
  u-q and f-p Static + Current Limitation : Subsystem
  Uref : Outport  VectorParamsAs1DForOutWhenUnconnected=off
  wires:
  Uabc_ref Generation max (m) = 1/1(Uabc_ref) -> Unit Delay/1
  Unit Delay/1 -> Uref/1
  I/1 -> PLL & Measurements/2(Iabc_prim)
  V/1 -> PLL & Measurements/1(Vabc_prim)
  PLL & Measurements/2(VdVq_prim) -> Current Regulator/1(VdVq_meas), u-q and f-p Static + Current Limitation/1(Voltage_dq [pu])
  Current Regulator/1(VdVq_conv) -> Uabc_ref Generation max (m) = 1/2(VdVq_conv)
  PLL & Measurements/1(wt) -> Uabc_ref Generation max (m) = 1/1(wt)
  Mux1/1 -> Saturation/1
  Saturation/1 -> Scope3/1
  PLL & Measurements/3(IdIq_prim) -> Current Regulator/2(IdIq_meas), Selector2/1, Selector/1
  Mux2/1 -> Saturation1/1
  Saturation1/1 -> Scope1/1
  u-q and f-p Static + Current Limitation/1(i_reflim_dq [pu]) -> Selector3/1, Selector1/1, Current Regulator/3(IdIq_ref)
  Selector/1 -> Mux1/2
  Selector1/1 -> Mux1/1
  Selector2/1 -> Mux2/2
  Selector3/1 -> Mux2/1
  PLL & Measurements/4(Freq) -> u-q and f-p Static + Current Limitation/2(Frequency [Hz])
  Converter Current Limit pu/1 -> u-q and f-p Static + Current Limitation/3(i_max[pu])

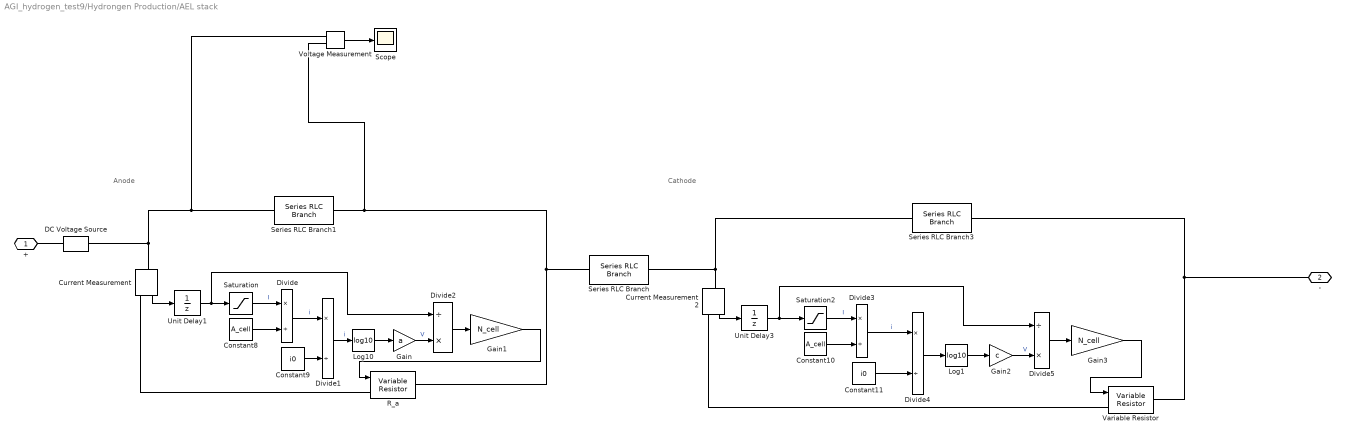
== system AGI_hydrogen_test9/Hydrongen Production/AEL stack ==
  note: Cathode
  note: Anode
  Constant10 : Constant  Value=A_cell
  Constant11 : Constant  Value=i0
  Constant8 : Constant  Value=A_cell
  Constant9 : Constant  Value=i0
  Current Measurement : spsCurrentMeasurementLib/Current Measurement  PhasorSimulation=off  OutputType=Complex  PSBequivalent=0
  Current Measurement2 : spsCurrentMeasurementLib/Current Measurement  PhasorSimulation=off  OutputType=Complex  PSBequivalent=0
  DC Voltage Source : spsDCVoltageSourceLib/DC Voltage Source  Amplitude=V_rev*N_cell  Measurements=None
  Divide{,1,3..4} (4 alike) : Product  Inputs=*/
  Divide2 : Product  Inputs=/*
  Divide5 : Product  Inputs=/*
  Gain : Gain  Gain=a
  Gain1 : Gain  Gain=N_cell
  Gain2 : Gain  Gain=c
  Gain3 : Gain  Gain=N_cell
  Log1 : Math  Operator=log10
  Log10 : Math  Operator=log10
  R_a : spsVariableResistorLib/Variable Resistor  Rabsmin=1e-3
  Saturation : Saturate  UpperLimit=inf  LowerLimit=1e-3
  Saturation2 : Saturate  UpperLimit=inf  LowerLimit=1e-3
  Scope : Scope
  Series RLC Branch : spsSeriesRLCBranchLib/Series RLC Branch  LConnTagsString=__new0  RConnTagsString=__new0  BranchType=R  Resistance=R_cell_ohm/A_cell*N_cell  Inductance=1e-3  SetiL0=off  InitialCurrent=0  Capacitance=1e-6  Setx0=off  InitialVoltage=0  Measurements=None
  Series RLC Branch1 : spsSeriesRLCBranchLib/Series RLC Branch  LConnTagsString=__new0  RConnTagsString=__new0  BranchType=C  Resistance=1  Inductance=1e-3  SetiL0=off  InitialCurrent=0  Capacitance=Ca*A_cell *1e-3/N_cell  Setx0=on  InitialVoltage=V0_a_cell*N_cell  Measurements=None
  Series RLC Branch3 : spsSeriesRLCBranchLib/Series RLC Branch  LConnTagsString=__new0  RConnTagsString=__new0  BranchType=C  Resistance=1  Inductance=1e-3  SetiL0=off  InitialCurrent=0  Capacitance=Cc*A_cell *1e-3/N_cell  Setx0=on  InitialVoltage=V0_a_cell*N_cell  Measurements=None
  Unit Delay1 : UnitDelay  InitialCondition=I0_a  SampleTime=-1  HasFrameUpgradeWarning=on
  Unit Delay3 : UnitDelay  InitialCondition=I0_c  SampleTime=-1  HasFrameUpgradeWarning=on
  Variable Resistor : spsVariableResistorLib/Variable Resistor  Rabsmin=1e-3
  Voltage Measurement : spsVoltageMeasurementLib/Voltage Measurement  PhasorSimulation=off  OutputType=Complex  PSBequivalent=0
  + : PMIOPort  Side=Left
  - : PMIOPort  Port=2  Side=Right
  wires:
  Saturation/1 -> Divide/1  "I"
  Constant8/1 -> Divide/2
  Gain/1 -> Divide2/2  "V"
  Gain1/1 -> R_a/1
  Divide2/1 -> Gain1/1
  Log10/1 -> Gain/1
  Current Measurement/1 -> Unit Delay1/1
  Current Measurement2/1 -> Unit Delay3/1
  Saturation2/1 -> Divide3/1  "I"
  Gain3/1 -> Variable Resistor/1
  Constant10/1 -> Divide3/2
  Divide5/1 -> Gain3/1
  Gain2/1 -> Divide5/2  "V"
  Divide4/1 -> Log1/1
  Log1/1 -> Gain2/1
  Constant11/1 -> Divide4/2
  Divide3/1 -> Divide4/1  "i"
  Divide/1 -> Divide1/1  "i"
  Constant9/1 -> Divide1/2
  Divide1/1 -> Log10/1  "i"
  Unit Delay1/1 -> Saturation/1, Divide2/1
  Unit Delay3/1 -> Divide5/1, Saturation2/1
  Voltage Measurement/1 -> Scope/1
  connections:
  R_a/RConn1 -- Voltage Measurement/LConn2 -- Series RLC Branch1/RConn1 -- Series RLC Branch/LConn1
  +/RConn1 -- DC Voltage Source/RConn1
  Current Measurement/RConn1 -- R_a/LConn1
  Series RLC Branch/RConn1 -- Current Measurement2/LConn1 -- Series RLC Branch3/LConn1
  Current Measurement2/RConn1 -- Variable Resistor/LConn1
  Series RLC Branch3/RConn1 -- -/RConn1 -- Variable Resistor/RConn1
  Voltage Measurement/LConn1 -- DC Voltage Source/LConn1 -- Current Measurement/LConn1 -- Series RLC Branch1/LConn1

== system AGI_hydrogen_test9/Hydrongen Production/VSC Control ==
  note: VSC Main Controller
  V : Inport  PortDimensions=3
  I : Inport  Port=2  PortDimensions=3
  Enable : EnablePort
  Constant : Constant  Value=-1
  Current Regulator : Subsystem
  Mux1 : Mux  Inputs=2
  PLL & Measurements : Subsystem
  Q in pu1 : Step  Time=2  After=0.5*0  SampleTime=0
  Uabc_ref Generation max (m) = 1 : Subsystem
  Unit Delay : UnitDelay  SampleTime=Ts_Control  HasFrameUpgradeWarning=on
  Uref : Outport  VectorParamsAs1DForOutWhenUnconnected=off
  wires:
  Uabc_ref Generation max (m) = 1/1(Uabc_ref) -> Unit Delay/1
  Unit Delay/1 -> Uref/1
  I/1 -> PLL & Measurements/2(Iabc_prim)
  V/1 -> PLL & Measurements/1(Vabc_prim)
  PLL & Measurements/2(VdVq_prim) -> Current Regulator/1(VdVq_meas)
  PLL & Measurements/3(IdIq_prim) -> Current Regulator/2(IdIq_meas)
  Current Regulator/1(VdVq_conv) -> Uabc_ref Generation max (m) = 1/2(VdVq_conv)
  PLL & Measurements/1(wt) -> Uabc_ref Generation max (m) = 1/1(wt)
  Q in pu1/1 -> Mux1/2
  Mux1/1 -> Current Regulator/3(IdIq_ref)  "idiq_ref"
  Constant/1 -> Mux1/1

== system AGI_hydrogen_test9/PV/DC//DC 1 ==
  m_PV : Inport
  P_limit : Inport  Port=2
  Boost Converter (Average Model) : Subsystem  mask(Boost Converter (Average Model)){Ts=Ts_Power}
      mask prompts: Ts "Sample time:"
      mask Display: disp('Boost\n(Average)')
  Bus Selector : BusSelector  OutputSignals=V_PV,I_PV
  Bus Selector1 : BusSelector  OutputSignals=V_PV,I_PV
  C : spsSeriesRLCBranchLib/Series RLC Branch  LConnTagsString=__new0  RConnTagsString=__new0  BranchType=C  Resistance=1.0  Inductance=1.0  SetiL0=off  InitialCurrent=0  Capacitance=100e-6  Setx0=on  InitialVoltage=260  Measurements=Branch voltage
  Eliminate algebric loop2 : UnitDelay  InitialCondition=0.485  SampleTime=Ts_Control  HasFrameUpgradeWarning=on
  L1 : spsSeriesRLCBranchLib/Series RLC Branch  LConnTagsString=__new0  RConnTagsString=__new0  BranchType=RL  Resistance=0.001  Inductance=5e-3  SetiL0=off  InitialCurrent=0  Capacitance=1e-6  Setx0=off  InitialVoltage=0  Measurements=None
  Logical Operator : Logic  Operator=NOT  AllPortsSameDT=off  OutDataTypeStr=boolean
  MPPT Parameters : Subsystem
  "MPPT Control  " : MATLAB Function  TreatAsAtomicUnit=on
  Mean : spsMeanLib/Mean  Freq=60  Vinit=100  Ts=Ts_Control
  Product : Product  RndMeth=Zero
  WkW : Gain  Gain=1/1000
  " +" : PMIOPort  Side=Right
  +PV : PMIOPort  Port=2  Side=Left
  -PV : PMIOPort  Port=3  Side=Left
  " -" : PMIOPort  Port=4  Side=Right
  tag scope: D1=global, Pmean1=global, m_PV1=global
  wires:
  "MPPT Control  "/1(D) -> Eliminate algebric loop2/1
  MPPT Parameters/1(Param) -> "MPPT Control  "/1(Param)
  Eliminate algebric loop2/1 -> Boost Converter (Average Model)/1(D), [D1]
  m_PV/1 -> Bus Selector1/1, [m_PV1], Bus Selector/1
  Bus Selector/1 -> "MPPT Control  "/3(V)  "<V_PV>"
  Bus Selector/2 -> "MPPT Control  "/4(I)  "<I_PV>"
  Bus Selector1/1 -> Product/1  "<V_PV>"
  Product/1 -> WkW/1
  Bus Selector1/2 -> Product/2  "<I_PV>"
  WkW/1 -> Mean/1  "Pmean_PV (kW)"
  Mean/1 -> [Pmean1]
  Boost Converter (Average Model)/1(Disable_MPPT) -> Logical Operator/1
  Logical Operator/1 -> "MPPT Control  "/2(Enabled)
  P_limit/1 -> Boost Converter (Average Model)/2(Plimit)
  connections:
  C/LConn1 -- +PV/RConn1 -- L1/LConn1
  L1/RConn1 -- Boost Converter (Average Model)/LConn1
  C/RConn1 -- Boost Converter (Average Model)/RConn2 -- " -"/RConn1 -- -PV/RConn1
  Boost Converter (Average Model)/RConn1 -- " +"/RConn1

== system AGI_hydrogen_test9/PV/VSC Control1 ==
  note: The q-u-static should be implemented here, using the Iq-ref value.
      | The p-f-static (overfrequency power reduction) must act directly on the PV-power to ensure the U-DC balance is kept.
  note: VSC Main Controller
  V : Inport  PortDimensions=3
  I : Inport  Port=2  PortDimensions=3
  Vdc : Inport  Port=3  PortDimensions=1
  Converter Current Limit pu : Constant  Value=1.5
  Current Regulator : Subsystem
  Demux : Demux  Outputs=2
  Mux : Mux  Inputs=2
  Mux1 : Mux  Inputs=2
  PLL & Measurements : Subsystem
  Scope{,1..4} (5 alike) : Scope
  Uabc_ref Generation max (m) = 1 : Subsystem
  Unit Delay : UnitDelay  SampleTime=Ts_Control  HasFrameUpgradeWarning=on
  VDC Regulator : Subsystem
  Vdc_ref1 : Constant  Value=Vdc_ref
  u-q and f-p Static + Current Limitation : Subsystem
  p_limit [pu] : Outport  VectorParamsAs1DForOutWhenUnconnected=off
  Uref : Outport  Port=2  VectorParamsAs1DForOutWhenUnconnected=off
  wires:
  Vdc_ref1/1 -> VDC Regulator/2(Vdc_ref)
  Uabc_ref Generation max (m) = 1/1(Uabc_ref) -> Unit Delay/1
  Unit Delay/1 -> Uref/1
  I/1 -> PLL & Measurements/2(Iabc_prim)
  V/1 -> PLL & Measurements/1(Vabc_prim)
  Vdc/1 -> Scope1/1, VDC Regulator/1(Vdc_meas)
  PLL & Measurements/2(VdVq_prim) -> u-q and f-p Static + Current Limitation/1(Voltage_dq [pu]), Scope2/1, Current Regulator/1(VdVq_meas)
  PLL & Measurements/3(IdIq_prim) -> Mux1/2, Current Regulator/2(IdIq_meas)
  Mux/1 -> Current Regulator/3(IdIq_ref)
  Current Regulator/1(VdVq_conv) -> Uabc_ref Generation max (m) = 1/2(VdVq_conv)
  PLL & Measurements/1(wt) -> Uabc_ref Generation max (m) = 1/1(wt)
  VDC Regulator/1(Id_ref) -> Scope/1, Mux/1
  u-q and f-p Static + Current Limitation/1(i_reflim_dq [pu]) -> Scope4/1, Mux1/1, Demux/1
  PLL & Measurements/4(Freq) -> u-q and f-p Static + Current Limitation/2(Frequency [Hz])
  Converter Current Limit pu/1 -> u-q and f-p Static + Current Limitation/3(i_max[pu])
  Mux1/1 -> Scope3/1
  Demux/2 -> Mux/2
  Demux/1 -> p_limit [pu]/1

== system AGI_hydrogen_test9/TestCases SimpleGrid1/Int ==
  In : Inport
  Constant6 : Constant  Value=2*pi
  Initial : InitialCondition  Value=0
  Integrator1 : Integrator  ExternalReset=rising  InitialConditionSource=external  InitialCondition=sps.Phase_Init*pi/180  ShowStatePort=on
  Relational Operator : RelationalOperator  Operator=>  OutDataTypeStr=boolean  InputSameDT=off
  Subtract : Sum  Inputs=+-
  Out : Outport
  wires:
  Integrator1/1 -> Out/1
  Initial/1 -> Integrator1/3
  In/1 -> Integrator1/1
  Relational Operator/1 -> Integrator1/2
  Subtract/1 -> Initial/1
  Integrator1/State -> Relational Operator/1, Subtract/1
  Constant6/1 -> Relational Operator/2, Subtract/2

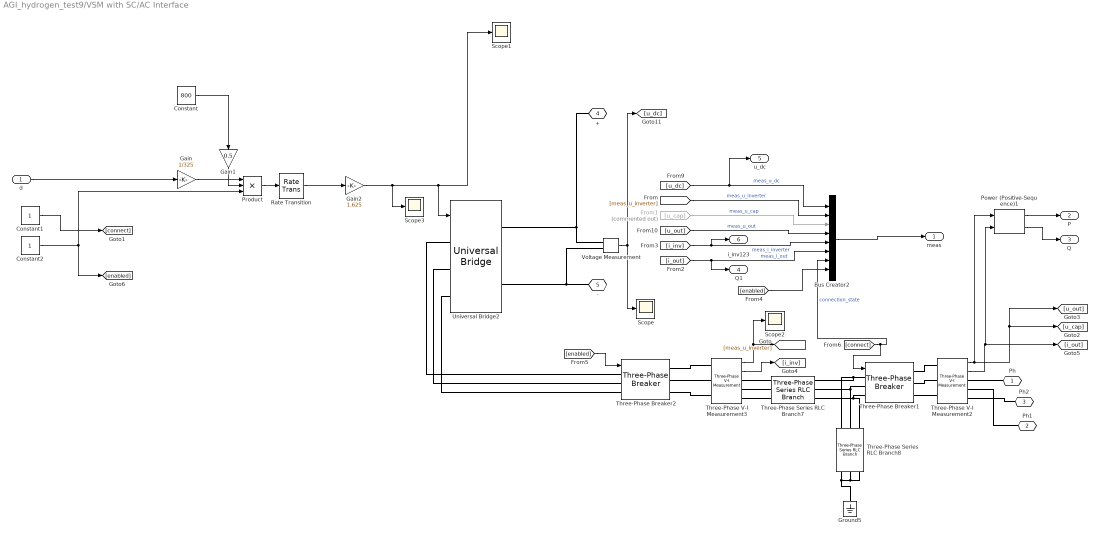
== system AGI_hydrogen_test9/VSM with SC/AC Interface ==
  d : Inport
  Bus Creator2 : BusCreator  Inputs=8
  Constant : Constant  Value=800
  Constant1 : Constant
  Constant2 : Constant
  From1 : From  Commented=on  GotoTag=u_cap
  Gain : Gain  Gain=1/325
  Gain1 : Gain  Gain=0.5
  Gain2 : Gain  Gain=1.625
  Ground5 : spsGroundLib/Ground  LConnTagsString=a
  Power (Positive-Sequence)1 : spsPowerPositiveSequenceLib/Power (Positive-Sequence)  Freq=50  Vinit=[20200 0]  Iinit=[12.3 0]  Ts=Ts_Control
  Product : Product  Inputs=3
  Rate Transition : RateTransition  Integrity=off  OutPortSampleTime=HWSampleTime
  Scope{,1..3} (4 alike) : Scope
  Three-Phase Series RLC Branch7 : spsThreePhaseSeriesRLCBranchLib/Three-Phase Series RLC Branch  LConnTagsString=A|B|C  RConnTagsString=A|B|C  BranchType=RL  Resistance=LCL.SI.R1  Inductance=LCL.SI.L1  Capacitance=1e-6  Measurements=None
  Three-Phase Series RLC Branch8 : spsThreePhaseSeriesRLCBranchLib/Three-Phase Series RLC Branch  LConnTagsString=A|B|C  RConnTagsString=A|B|C  BranchType=RC  Resistance=LCL.SI.Rc  Inductance=Grid.SI.L  Capacitance=LCL.SI.C  Measurements=None
  Three-Phase V-I Measurement2 : spsThreePhaseVIMeasurementLib/Three-Phase V-I Measurement  VoltageMeasurement=phase-to-ground  SetLabelV=off  LabelV=Vabc  Vpu=off  VpuLL=off  CurrentMeasurement=yes  SetLabelI=off  LabelI=Iabc  Ipu=off  Pbase=100e6  Vbase=500e3  OutputType=Complex  PhasorSimulation=off  PSBequivalent=0
  Three-Phase V-I Measurement3 : spsThreePhaseVIMeasurementLib/Three-Phase V-I Measurement  VoltageMeasurement=phase-to-ground  SetLabelV=off  LabelV=Vabc  Vpu=off  VpuLL=off  CurrentMeasurement=yes  SetLabelI=off  LabelI=Iabc  Ipu=off  Pbase=100e6  Vbase=500e3  OutputType=Complex  PhasorSimulation=off  PSBequivalent=0
  Three-Phase Breaker1 : spsThreePhaseBreakerLib/Three-Phase Breaker  InitialState=open  SwitchA=on  SwitchB=on  SwitchC=on  SwitchTimes="[1/60  5/60]"  External=on  BreakerResistance=1e-6  SnubberResistance=1e6  SnubberCapacitance=inf  Measurements=None
  Three-Phase Breaker2 : spsThreePhaseBreakerLib/Three-Phase Breaker  InitialState=open  SwitchA=on  SwitchB=on  SwitchC=on  SwitchTimes="[1/60  5/60]"  External=on  BreakerResistance=1e-6  SnubberResistance=1e6  SnubberCapacitance=inf  Measurements=None
  Universal Bridge2 : spsUniversalBridgeLib/Universal Bridge  Arms=3  SnubberResistance=1e5  SnubberCapacitance=inf  Device=Average-model based VSC  Ron=1e-3  Lon=0  ForwardVoltages="[  0  0  ]"  ForwardVoltage=0  GTOparameters=[ 10e-6 , 20e-6 ]  IGBTparameters=[ 1e-6 , 2e-6 ]  Measurements=None  Measurements_2=None  converterType=Rectifier
  Voltage Measurement : spsVoltageMeasurementLib/Voltage Measurement  PhasorSimulation=off  OutputType=Complex  PSBequivalent=0
  Ph : PMIOPort  Side=Right
  Ph1 : PMIOPort  Port=2  Side=Right
  Ph2 : PMIOPort  Port=3  Side=Right
  + : PMIOPort  Tag=PMCPort  Port=4  Side=Right
  - : PMIOPort  Tag=PMCPort  Port=5  Side=Right
  meas : Outport
  P : Outport  Port=2
  Q : Outport  Port=3
  Q1 : Outport  Port=4
  u_dc : Outport  Port=5
  i_inv123 : Outport  Port=6
  wires:
  [meas_u_inverter] -> Bus Creator2/2  "meas_u_inverter"
  [connect] -> Bus Creator2/7, Three-Phase Breaker1/1  "connection_state"
  From1/1 -> Bus Creator2/3  "meas_u_cap"
  Constant1/1 -> [connect]
  [i_out] -> Q1/1, Bus Creator2/6  "meas_i_out"
  Three-Phase V-I Measurement2/1 -> Power (Positive-Sequence)1/1, [u_cap], [u_out]
  Three-Phase V-I Measurement3/2 -> [i_inv]
  [i_inv] -> i_inv123/1, Bus Creator2/5  "meas_i_inverter"
  Constant2/1 -> Product/3, [enabled]
  [u_out] -> Bus Creator2/4  "meas_u_out"
  Product/1 -> Rate Transition/1
  [u_dc] -> u_dc/1, Bus Creator2/1  "meas_u_dc"
  Three-Phase V-I Measurement2/2 -> Power (Positive-Sequence)1/2, [i_out]
  Three-Phase V-I Measurement3/1 -> Scope2/1, [meas_u_inverter]
  Gain1/1 -> Product/2
  Bus Creator2/1 -> meas/1
  d/1 -> Gain/1
  [enabled] -> Bus Creator2/8
  [enabled] -> Three-Phase Breaker2/1
  Rate Transition/1 -> Gain2/1
  Gain/1 -> Product/1
  Power (Positive-Sequence)1/1 -> P/1
  Power (Positive-Sequence)1/2 -> Q/1
  Voltage Measurement/1 -> Scope/1, [u_dc]
  Constant/1 -> Gain1/1
  Gain2/1 -> Scope3/1, Scope1/1, Universal Bridge2/1
  connections:
  Three-Phase Series RLC Branch8/RConn2 -- Ground5/LConn1 -- Three-Phase Series RLC Branch8/RConn1 -- Three-Phase Series RLC Branch8/RConn3
  Three-Phase V-I Measurement3/RConn1 -- Three-Phase Series RLC Branch7/LConn1
  Three-Phase Series RLC Branch8/LConn1 -- Three-Phase Breaker1/LConn1 -- Three-Phase Series RLC Branch7/RConn1
  Three-Phase Series RLC Branch7/RConn2 -- Three-Phase Breaker1/LConn2 -- Three-Phase Series RLC Branch8/LConn2
  Three-Phase Breaker1/RConn1 -- Three-Phase V-I Measurement2/LConn1
  Three-Phase Series RLC Branch7/RConn3 -- Three-Phase Breaker1/LConn3 -- Three-Phase Series RLC Branch8/LConn3
  Three-Phase V-I Measurement3/RConn2 -- Three-Phase Series RLC Branch7/LConn2
  Three-Phase V-I Measurement2/RConn3 -- Ph2/RConn1
  Ph/RConn1 -- Three-Phase V-I Measurement2/RConn1
  Three-Phase Breaker1/RConn2 -- Three-Phase V-I Measurement2/LConn2
  Three-Phase V-I Measurement3/RConn3 -- Three-Phase Series RLC Branch7/LConn3
  Three-Phase Breaker1/RConn3 -- Three-Phase V-I Measurement2/LConn3
  Three-Phase V-I Measurement2/RConn2 -- Ph1/RConn1
  Three-Phase Breaker2/RConn2 -- Three-Phase V-I Measurement3/LConn2
  Three-Phase Breaker2/RConn1 -- Three-Phase V-I Measurement3/LConn1
  Three-Phase Breaker2/RConn3 -- Three-Phase V-I Measurement3/LConn3
  +/RConn1 -- Voltage Measurement/LConn1 -- Universal Bridge2/RConn1
  Universal Bridge2/LConn2 -- Three-Phase Breaker2/LConn2
  -/RConn1 -- Voltage Measurement/LConn2 -- Universal Bridge2/RConn2
  Universal Bridge2/LConn1 -- Three-Phase Breaker2/LConn1
  Three-Phase Breaker2/LConn3 -- Universal Bridge2/LConn3
